simulink model "DSPBA_design_template"  (Simulink 7.5)
settings: Solver=FixedStepDiscrete  StartTime=0.0  StopTime=my_design.endTime  RelTol=1e-3
PreLoadFcn:
  | % Run the setup script when the model is opened
  | setup_DSPBA_design_template;
InitFcn:
  | % Run the setup script again just before the
  | % model is run, so that any updates made
  | % after opening are applied.
  | setup_DSPBA_design_template;
undefined symbols (not defined in the file or in its folder): AdvDSPBChannelOutDisplay, dspba_ChannelInVis, dspba_ChannelOutVis, dspba_internal_get_channel_ports, latency, my_design
libraries: DSPBABase x7, DSPBAPrim x3, DSPBAUtilities x2, DSPBAFilters x1
settings Model: Creator=mjervis  LastModifiedBy=mjervis
settings DebuggingCC: InheritedTsInSrcMsg=none

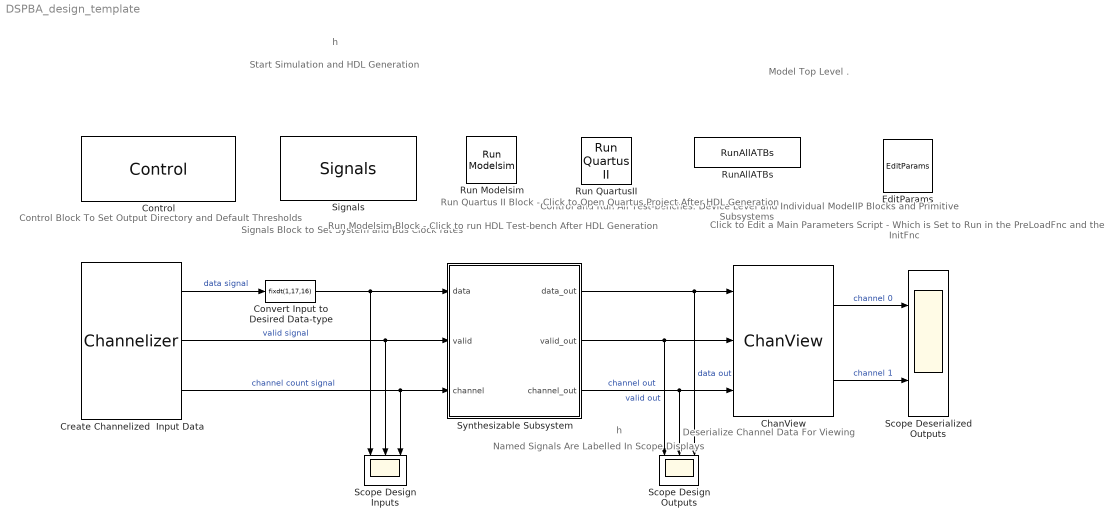
== system DSPBA_design_template ==
  note: h
  note: Start Simulation and
      | HDL Generation
  note: Control and Run All
      | Test-benches: Device
      | Level and Individual
      | ModelIP Blocks and
      | Primitive Subsystems
  note: Model Top Level
      |                                               .
  note: Control Block To Set Output
      | Directory and Default Thresholds
  note: Signals Block to Set System
      | and Bus Clock rates
  note: Run Modelsim
      | Block - Click to run
      | HDL Test-bench After
      | HDL Generation
  note: Run Quartus II
      | Block - Click to Open
      | Quartus Project After
      | HDL Generation
  note: Click to Edit a Main Parameters
      | Script - Which is Set to Run in the
      | PreLoadFnc and the InitFnc
  note: h
  note: Named Signals
      | Are Labelled In
      | Scope Displays
  note: Deserialize Channel
      | Data For Viewing
  ChanView : DSPBABase/ChanView  nchans=my_design.ChanCount  chan_vector=[0:1]  latency=2  version=20090407
  Control : DSPBABase/Control  generate=on  destination=./rtl  language=VHDL  autotestbench=on  signaldepth=2  coveragetestbench=off  logs=off  spacewidth=2  spacenum=1  addrwidth=10  datawidth=16  dataendian=Big Endian  hierarchicalnames=off  ramThresholdBits=-1  distRamThresholdBits=-1  mlabThresholdBits=-1  hardMultiplierThresholdLuts=-1  version=20090407
  Convert Input to Desired Data-type : DataTypeConversion  OutDataTypeMode=Specify via dialog  OutDataType=fixdt(1,17,16)  OutDataTypeStr=fixdt(1,17,16)  SaturateOnIntegerOverflow=on
  Create Channelized  Input Data : DSPBAUtilities/Channelizer  SystemSampleTime=-1  data_input=my_design.inputdata  folding=my_design.Period  samples_valid=my_design.ChanCycleCount  samples_idle=my_design.Period-my_design.ChanCycleCount
  EditParams : DSPBABase/EditParams  SystemSampleTime=-1  version=20090407
  Run Modelsim : DSPBABase/Run Modelsim  SystemSampleTime=-1  version=20090407
  "Run QuartusII " : DSPBABase/Run Quartus II  SystemSampleTime=-1  version=20090407
  RunAllATBs : DSPBAUtilities/RunAllATBs  Description=|  SystemSampleTime=-1  version=20090407  runAllATBs=off  runSimulation=off  runFit=on  runDeviceLevelATB=off  openUI=off  warnOnChanMismatch=off  warnOnGPIOMismatch=on  runQuickModelCheck=off  exportDeviceOutput=on
      | Run run_modelsim_atb for each automatic test-bench (atb) created for the model                                                                                             
      |                                                                                                                                                                            
      | Example uses: run_all_atbs('demo_agc');                                                                                                                                    
      |                 run_all_atbs('demo_agc', true);                                                                                                                            
      |                 run_all_atbs('demo_agc', false, true);                                                                                                                     
      |                 run_all_atbs('demo_agc', true,  true);                                                                                                                     
      |                                                                                                                                                                            
      | Parameters: 	                                                                                                                                                              
      | model - name (string) of mdl file                             run_simulation	- run the simulation first?                                                                   
      | run_fit - run Quartus II?                                                                                                                                                  
      |                                                                                                                                                                            
      | Returns 1 if all tests were successful, 0 otherwise                                                                                                                        
      |                                                                                                                                                                            
      |  For the last option, when Quartus is run, it will tell you whether the fMax was met e.g.                                                                                  
      |        "Met FMax Requirement (FMax(220.17) >= Required(200))"                                                                                                              
      |                                                                                                                                                                            
      | Output is written to the Matlab Command window. In addition the results are written  to results.txt. An example results.txt, (which includes a failure for illustration) is
      |                                                                                                                                                                            
      | Starting demo_ifft_4096_natural Tests at 2008-12-23 15:32:52                                                                                                               
      | demo_ifft:  demo_ifft/FFT_4K_n/BitReverseCore hardware matches simulation (atb#1): PASSED                                                                                  
      | demo_ifft:  demo_ifft/FFT_4K_n/FFT_4K_Natural_BR hardware mismatches simulation (atb#2): FAILED                                                                            
      | demo_ifft:  Quartus II compilation was successful. (Directory=../quartus_demo_ifft_FFT_4K_n_1): PASSED                                                                     
      | demo_ifft:  Met FMax Requirement (FMax(220.17) >= Required(200)): PASSED                                                                                                   
      | Finished demo_ifft Tests at 2008-12-23 15:45:45 (4 Tests, 3 Passes, 0 Skipped, 0 Failed (fmax), 1 Failed (non-fmax)
  Scope Deserialized Outputs : Scope  NumInputPorts=2
      settings: TimeRange=100  YMin=-0.2~-0.25  YMax=0.5~0.25  SaveName=ScopeData2  DataFormat=Array
  Scope Design Inputs : Scope  NumInputPorts=3
      settings: TimeRange=100  YMin=-1~0~0  YMax=1~2~3  DataFormat=Array
  Scope Design Outputs : Scope  NumInputPorts=3
      settings: TimeRange=100  YMin=0~0~-0.4  YMax=1~1~0.6  DataFormat=Array
  Signals : DSPBABase/Signals  SystemSampleTime=-1  clk=clk  freq=my_design.ClockRate  margin=my_design.ClockMargin  rst=areset  rstactive=High  bus=bus  enbusclock=off  busfreq=200  bussync=off  version=20090407
  Synthesizable Subsystem : Subsystem
  wires:
  Synthesizable Subsystem/2(valid_out) -> Scope Design Outputs/1, ChanView/2  "valid out"
  Synthesizable Subsystem/3(channel_out) -> Scope Design Outputs/2, ChanView/3  "channel out"
  Synthesizable Subsystem/1(data_out) -> Scope Design Outputs/3, ChanView/1  "data out"
  Create Channelized  Input Data/1 -> Convert Input to Desired Data-type/1  "data signal"
  Create Channelized  Input Data/2 -> Synthesizable Subsystem/2(valid), Scope Design Inputs/2  "valid signal"
  Create Channelized  Input Data/3 -> Synthesizable Subsystem/3(channel), Scope Design Inputs/3  "channel count signal"
  Convert Input to Desired Data-type/1 -> Synthesizable Subsystem/1(data), Scope Design Inputs/1
  ChanView/1 -> Scope Deserialized Outputs/1  "channel 0"
  ChanView/2 -> Scope Deserialized Outputs/2  "channel 1"

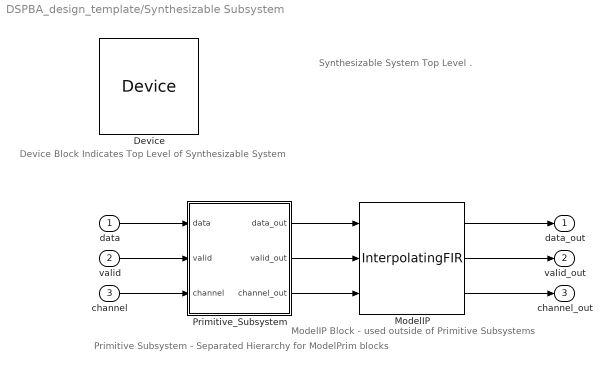
== system DSPBA_design_template/Synthesizable Subsystem ==
  note: Synthesizable System Top Level
      |                                                                   .
  note: Device Block Indicates
      | Top Level of Synthesizable
      | System
  note: ModelIP Block - used
      | outside of Primitive
      | Subsystems
  note: Primitive Subsystem -
      | Separated Hierarchy for
      | ModelPrim blocks
  data : Inport
  valid : Inport  Port=2
  channel : Inport  Port=3
  Device : DSPBABase/Device  SystemSampleTime=-1  family=Stratix V  deviceMember=Stratix V GX  stratix4device=Stratix IV E  hardcopy4device=HardCopy IV E  stratix5device=Stratix V GX  device=AUTO  speed=-3  stratixSpeed=-5  stratix2Speed=-3  stratix3Speed=-2  stratix4gxSpeed=-2  stratix4gtSpeed=-1  cyclone2Speed=-6  cyclone3Speed=-7  arria2Speed=-4  cyclone4eSpeed=-8  stratix5Speed=-3  arria5Speed=-4  arriaSpeed=-6  cyclone3lsSpeed=-7  cyclone5Speed=-6  ecp2Speed=-7  hardcopycompat=off  version=20110729
  ModelIP : DSPBAFilters/InterpolatingFIR  nInputRate=my_design.filter1.SampleRate  interp=my_design.filter1.Interpolation  nchan=my_design.ChanCount  symmetry=Symmetrical  coef=fi(fir1(my_design.filter1.FilterLength, 0.5 ),1,16,15)  addr=512  rwmode=Write  nband=Use All Taps  latency=6  version=20090407
  Primitive_Subsystem : Subsystem
  data_out : Outport
  valid_out : Outport  Port=2
  channel_out : Outport  Port=3
  wires:
  data/1 -> Primitive_Subsystem/1(data)
  valid/1 -> Primitive_Subsystem/2(valid)
  Primitive_Subsystem/2(valid_out) -> ModelIP/2
  channel/1 -> Primitive_Subsystem/3(channel)
  Primitive_Subsystem/3(channel_out) -> ModelIP/3
  Primitive_Subsystem/1(data_out) -> ModelIP/1
  ModelIP/1 -> data_out/1
  ModelIP/2 -> valid_out/1
  ModelIP/3 -> channel_out/1

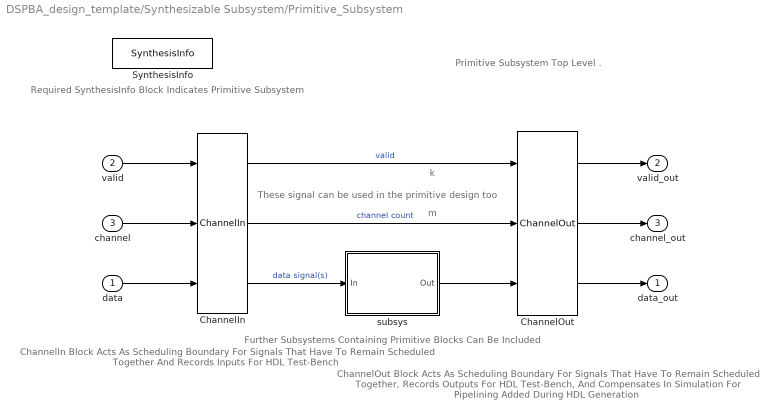
== system DSPBA_design_template/Synthesizable Subsystem/Primitive_Subsystem ==
  note: Primitive Subsystem Top Level
      |                                                                   .
  note: ChannelIn Block
      | Acts As Scheduling
      | Boundary For Signals
      | That Have To Remain
      | Scheduled Together And
      | Records Inputs For HDL
      | Test-Bench
  note: Further Subsystems Containing
      | Primitive Blocks Can Be Included
  note: ChannelOut Block
      | Acts As Scheduling
      | Boundary For Signals
      | That Have To Remain
      | Scheduled Together,
      | Records Outputs For HDL
      | Test-Bench, And Compensates
      | In Simulation For Pipelining
      | Added During HDL Generation
  note: Required SynthesisInfo
      | Block Indicates Primitive
      | Subsystem
  note: These signal can
      | be used in the
      | primitive design too
  note: k
  note: m
  data : Inport
  valid : Inport  Port=2
  channel : Inport  Port=3
  ChannelIn : DSPBAPrim/ChannelIn  primtype=channelin  nInputs=dspba_internal_get_channel_ports(gcb)  nOutputs=dspba_internal_get_channel_ports(gcb)  omode=Inherit via internal rule  otype=sfix(16)  scale=2^-15  rndmethod=Unbiased  factor=1  satmethod=Symmetric  shift_vec=[0 1 2 -1]  value=1  inPortNames=['v'; 'c'; '0'; '1'; '2'; '3'; '4'; '5'; '6'; '7'; '8'; '9'; 'A'; 'B'; 'D'; 'E'; 'F'; 'G'; 'H'; 'I'; 'J'; 'K'; 'L'; 'M'; 'N'; 'O'; 'P'; 'Q'; 'R'; 'S'; 'T'; 'U'; 'W'; 'X'; 'Y'; 'Z']  outPortNames=['v'; 'c'; '0'; '1'; '2'; '3'; '4'; '5'; '6'; '7'; '8'; '9'; 'A'; 'B'; 'D'; 'E'; 'F'; 'G'; 'H'; 'I'; 'J'; 'K'; 'L'; 'M'; 'N'; 'O'; 'P'; 'Q'; 'R'; 'S'; 'T'; 'U'; 'W'; 'X'; 'Y'; 'Z']  dspbaimage=dspba_prim.jpg  text=fprintf('In');  style=Optimised  dataSignals=1  foldingEnabled=off  channels=1  sampleRate=200  visibilities=dspba_ChannelInVis(gcb)  version=20090408
  ChannelOut : DSPBAPrim/ChannelOut  primtype=channelout  nInputs=dspba_internal_get_channel_ports(gcb)  nOutputs=dspba_internal_get_channel_ports(gcb)  omode=Inherit via internal rule  otype=sfix(16)  scale=2^-15  rndmethod=Unbiased  factor=1  satmethod=Symmetric  shift_vec=[0 1 2 -1]  value=1  inPortNames=['v'; 'c'; '0'; '1'; '2'; '3'; '4'; '5'; '6'; '7'; '8'; '9'; 'A'; 'B'; 'D'; 'E'; 'F'; 'G'; 'H'; 'I'; 'J'; 'K'; 'L'; 'M'; 'N'; 'O'; 'P'; 'Q'; 'R'; 'S'; 'T'; 'U'; 'W'; 'X'; 'Y'; 'Z']  outPortNames=['v'; 'c'; '0'; '1'; '2'; '3'; '4'; '5'; '6'; '7'; '8'; '9'; 'A'; 'B'; 'D'; 'E'; 'F'; 'G'; 'H'; 'I'; 'J'; 'K'; 'L'; 'M'; 'N'; 'O'; 'P'; 'Q'; 'R'; 'S'; 'T'; 'U'; 'W'; 'X'; 'Y'; 'Z']  dspbaimage=dspba_prim.jpg  text=fprintf('Out%s', AdvDSPBChannelOutDisplay(latency));  style=Optimised  dataSignals=1  foldingEnabled=off  channels=1  sampleRate=200  visibilities=dspba_ChannelOutVis(gcb)  latency=0  version=20090408
  SynthesisInfo : DSPBAPrim/SynthesisInfo  primtype=synthinfo  nInputs=0  nOutputs=0  omode=Inherit via internal rule  otype=sfix(16)  scale=2^-15  rndmethod=Truncate  factor=1  satmethod=Symmetric  shift_vec=[0 1 2 -1]  value=99  inPortNames=[' '; ' ';]  outPortNames=[' ']  dspbaimage=dspba_prim_ctrl.jpg  text=fprintf('Style=%s', style);  style=Scheduled  visibilities=32768  constraintInUse=off  constraintRelation=>  constraintLimit=2  version=20090407
  subsys : Subsystem
  data_out : Outport
  valid_out : Outport  Port=2
  channel_out : Outport  Port=3
  wires:
  ChannelOut/3 -> data_out/1
  ChannelOut/2 -> channel_out/1
  ChannelOut/1 -> valid_out/1
  data/1 -> ChannelIn/3
  channel/1 -> ChannelIn/2
  valid/1 -> ChannelIn/1
  ChannelIn/1 -> ChannelOut/1  "valid"
  ChannelIn/2 -> ChannelOut/2  "channel count"
  ChannelIn/3 -> subsys/1(In)  "data signal(s)"
  subsys/1(Out) -> ChannelOut/3

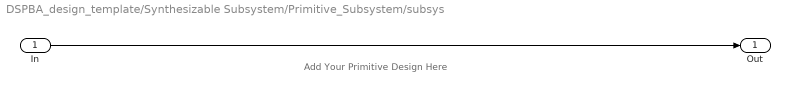
== system DSPBA_design_template/Synthesizable Subsystem/Primitive_Subsystem/subsys ==
  note: Add Your Primitive Design Here
  In : Inport
  Out : Outport
  wires:
  In/1 -> Out/1
